simulink model "part2"  (R2018a)
settings: Solver=VariableStepAuto  StartTime=0.0  StopTime=20  RelTol=1e-3
undefined symbols (not defined in the file or in its folder): gc, m
settings Model: Creator=jschm  LastModifiedBy=jschm

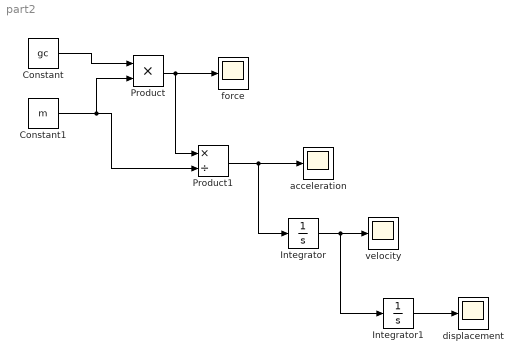
== system part2 ==
  "Constant " : Constant  Value=gc
  Constant1 : Constant  Value=m
  Integrator : Integrator  InitialCondition=200
  Integrator1 : Integrator  InitialCondition=10
  Product : Product
  Product1 : Product  Inputs=*/
  acceleration : Scope
  displacement : Scope
  force : Scope
  velocity : Scope
  wires:
  "Constant "/1 -> Product/1
  Product/1 -> Product1/1, force/1
  Constant1/1 -> Product/2, Product1/2
  Product1/1 -> Integrator/1, acceleration/1
  Integrator/1 -> Integrator1/1, velocity/1
  Integrator1/1 -> displacement/1
